simulink model "test_phase_shift_filter"  (R2025b)
settings: Solver=ode1  StartTime=0.0  StopTime=0.2  FixedStep=ts_inv  RelTol=1e-3
values from neighbouring files (symbols this model uses):
  freq = [0:1/u1:Nfft/2/u1-1/u1]'    [plotting_results_sim_results_30Hz_10kHz_1.m]    (also in plotting_results_sim_results_400Hz_10kHz_1.m; plotting_results_sim_results_400Hz_20kHz_1.m; plotting_results_sim_results_50Hz_10kHz_1.m; plotting_results_sim_results_50Hz_20kHz_1.m)
libraries: phase_shift_filter x1
settings Model: Creator=dbagn  LastModifiedBy=dbagn

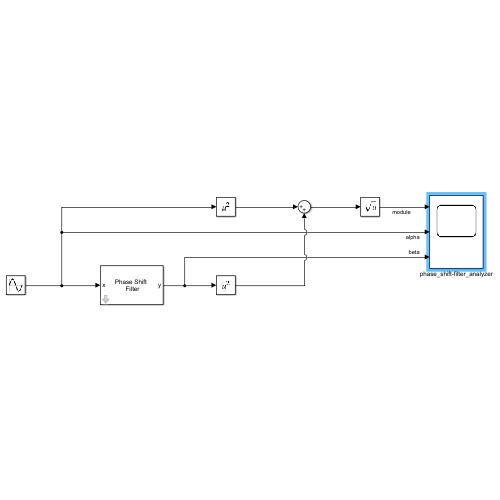
[thumbnail: Simulink's stored preview of the top-level diagram]
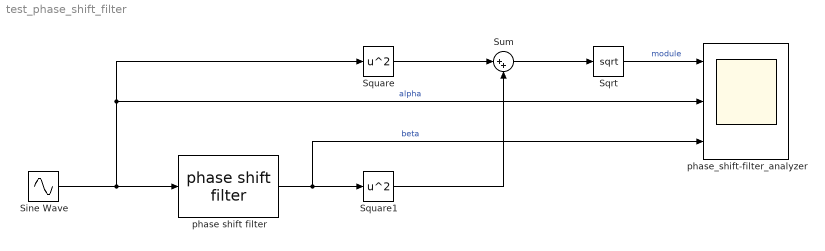
== system test_phase_shift_filter ==
  Sine Wave : Sin  Frequency=freq*2*pi  SampleTime=0
  Sqrt : Sqrt
  Square : Math  Operator=square
  Square1 : Math  Operator=square
  Sum : Sum  Inputs=|++
  phase shift filter : phase_shift_filter/phase shift filter  f=freq  scaling_factor=0.985-0.085/350*(freq-50)  ts=ts_inv
  phase_shift-filter_analyzer : Scope  NumInputPorts=3
      settings: SampleTime=ts_inv  ActiveDisplayYMinimum=-1.1297586136004538  ActiveDisplayYMaximum=1.507573484556453
  wires:
  Sine Wave/1 -> Square/1, phase_shift-filter_analyzer/2, phase shift filter/1  "alpha"
  phase shift filter/1 -> phase_shift-filter_analyzer/3, Square1/1  "beta"
  Square/1 -> Sum/1
  Square1/1 -> Sum/2
  Sum/1 -> Sqrt/1
  Sqrt/1 -> phase_shift-filter_analyzer/1  "module"
